simulink model "block_pendulum_discrete"  (Simulink 7.8)
settings: Solver=FixedStepDiscrete  StartTime=0.0  StopTime=inf  FixedStep=0.001  RelTol=1e-3
settings Model: Creator=imac  LastModifiedBy=aitor
settings DebuggingCC: FcnCallInpInsideContextMsg=Use local settings

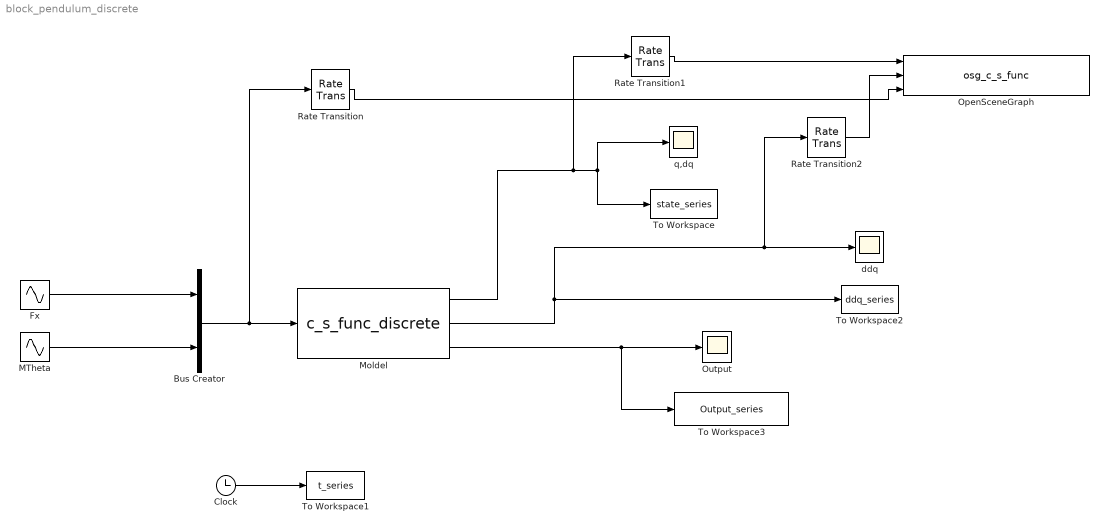
== system block_pendulum_discrete ==
  Bus Creator : BusCreator  Inputs=2
  Clock : Clock
  Fx : Sin  Amplitude=0  Frequency=0  Phase=pi/2  SampleTime=0
  MTheta : Sin  Amplitude=0  Frequency=0  Phase=pi/2  SampleTime=0
  Moldel : S-Function  FunctionName=c_s_func_discrete  Parameters=q dq param Delta_t  EnableBusSupport=off
      mask Type: S-function: mycsfunc
      mask Description: This is a S-function that does the continuous state space system.
      mask Display: disp('[M , Phi_q''] [ddq]\n[Phi_q , 0] [lambda]\n=\n [Q ] \n   [gamma] ');
  OpenSceneGraph : S-Function  FunctionName=osg_c_s_func  Parameters=param  EnableBusSupport=off
  Output : Scope
      settings: YMin=-1750  YMax=1000  SaveName=ScopeData2  SampleInput=on
  Rate Transition : RateTransition  OutPortSampleTime=0.01
  Rate Transition1 : RateTransition  OutPortSampleTime=0.01
  Rate Transition2 : RateTransition  OutPortSampleTime=0.01
  To Workspace : ToWorkspace  VariableName=state_series  SampleTime=-1  SaveFormat=Array
  To Workspace1 : ToWorkspace  VariableName=t_series  SampleTime=-1  SaveFormat=Array
  To Workspace2 : ToWorkspace  VariableName=ddq_series  SampleTime=-1  SaveFormat=Array
  To Workspace3 : ToWorkspace  VariableName=Output_series  SampleTime=-1  SaveFormat=Array
  ddq : Scope
      settings: YMin=-500  YMax=300  SampleInput=on
  q,dq : Scope
      settings: YMin=-0.03  YMax=0.17  SampleInput=on
  wires:
  Clock/1 -> To Workspace1/1
  Moldel/1 -> q,dq/1, To Workspace/1, Rate Transition1/1
  Moldel/2 -> To Workspace2/1, ddq/1, Rate Transition2/1
  Moldel/3 -> Output/1, To Workspace3/1
  Bus Creator/1 -> Moldel/1, Rate Transition/1
  MTheta/1 -> Bus Creator/2
  Fx/1 -> Bus Creator/1
  Rate Transition1/1 -> OpenSceneGraph/1
  Rate Transition2/1 -> OpenSceneGraph/2
  Rate Transition/1 -> OpenSceneGraph/3
